simulink library "tqd"  (R2021b)
settings: Solver=VariableStepAuto  StartTime=0.0  StopTime=10.0  RelTol=1e-3
undefined symbols (not defined in the file or in its folder): ATQD_BOSEnBPSPosn_X_kph, ATQD_BOSMap_X_rpm, ATQD_BOSMap_Y_pct, ATQD_CreepBaseTqD_X_kph, ATQD_CreepBaseTqD_Y_Deg, ATQD_CreepBaseTqR_X_kph, ATQD_CreepBaseTqR_Y_Deg, ATQD_CreepBPSDisPosn_X_Deg, ATQD_CreepBPSDisPosnR_X_Deg, ATQD_CreepBPSEnPosn_X_Deg, ATQD_CreepBPSEnPosnR_X_Deg, ATQD_CreepDeltaTq_X_kph, ATQD_CreepIterm_X_kph, ATQD_CreepIterm_Y_kph, ATQD_CreepItermMaxLimit_X_pct, ATQD_CreepPreloadTime_X_kph, ATQD_CreepPreloadTq_X_kph, ATQD_CreepPreloadTq_Y_s, ATQD_CreepProtTq_X_Deg, ATQD_CreepPterm_X_kph, ATQD_ECOTqMapD_X_rpm, ATQD_ECOTqMapD_Y_pct, ATQD_NL1TqMapD_X_rpm, ATQD_NL1TqMapD_Y_pct, ATQD_NRMRrEDUSpRat_X_rpm, ATQD_NRMRrEDUSpRat_Y_Nm, ATQD_PedalMapClimbUpLim_X_rpm, ATQD_PedalMapClimbUpLim_Y_Deg, ATQD_PreLoadTq_X_s, ATQD_SL1TqMapD_X_rpm, ATQD_SL1TqMapD_Y_pct, ATQD_WhlTqCapMotGain_X_pct, ATQD_WhlTqCapMotGain_Y_mV, ENUM_ACCPEDALLOWSW_LOWIDLE, ENUM_ACCPEDALLOWSW_NOIDLE, ENUM_CHRGPLUGSTA_NONE, ENUM_CRASHSTATE_NOCRASH, ENUM_DCDCFAULTSTA_WORKING, ENUM_DRIVEMODE_ECO, ENUM_DRIVEMODE_NRM, ENUM_DRIVEMODE_SPORT, ENUM_DRIVETRAIN_AWD, ENUM_DRIVETRAIN_FWD, ENUM_DRIVETRAIN_RWD, ENUM_EBSBRKSW_PRESSED, ENUM_EBSTORQUERWQ_LIMIT, ENUM_EBSTORQUERWQ_TORQUE, ENUM_EMTRQMODE_ACCL, ENUM_EMTRQMODE_BRAKING, ENUM_EMTRQMODE_COASTING, ENUM_EPBERROR_NORMAL, ENUM_EPBSTA_APPLIED, ENUM_EPBSTA_RELEASED, ENUM_EPBSTA_UNKNOWN, ENUM_EPBSTARAW_NOTSET, ENUM_EPBSTARAW_SET, ENUM_GEARACTUALPOSN_D, ENUM_GEARACTUALPOSN_N, ENUM_GEARACTUALPOSN_P, ENUM_GEARACTUALPOSN_R ... (+201)
libraries: hcu_lib x19, simulink x12
(part 1 of 6)
settings Model: Creator=13615  LastModifiedBy=FVT22063
settings SolverCC: AlgebraicLoopSolver=TrustRegion
settings DataIOCC: SaveFormat=Array  SignalLoggingSaveFormat=ModelDataLogs  ReturnWorkspaceOutputs=off
settings OptimizationCC: BlockReduction=off  BooleanDataType=off
settings DebuggingCC: SaveWithParameterizedLinksMsg=none  UnderspecifiedInitializationDetection=Classic  MergeDetectMultiDrivingBlocksExec=none  SignalResolutionControl=TryResolveAllWithWarning
settings HardwareCC: TargetUnknown=on
settings ModelReferenceCC: PropagateSignalLabelsOutOfModel=off
settings SFSimCC: SimUseLocalCustomCode=off
settings RTWCC: RTWUseLocalCustomCode=off
settings ConfigComp: CovMetricSettings=dw  CovSaveCumulativeToWorkspaceVar=on  CovSaveSingleToWorkspaceVar=on

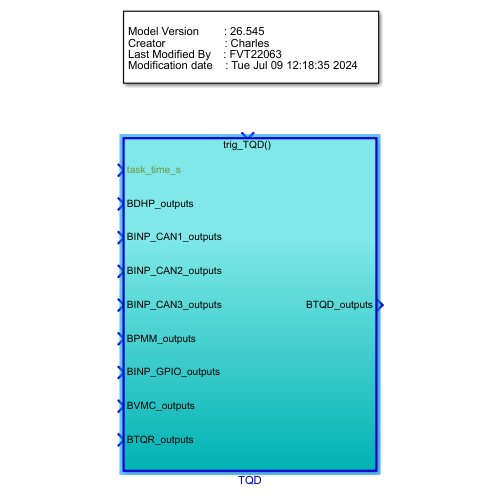
[thumbnail: Simulink's stored preview of the top-level diagram]
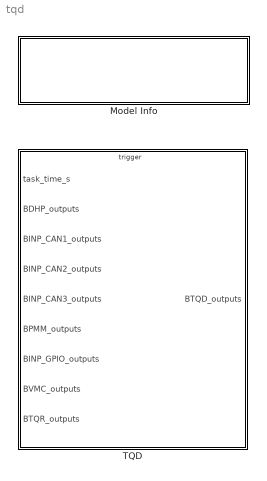
== system tqd ==
  Model Info : Subsystem  LoadFcn=slcm LoadBlock;  InitFcn=slcm('UpdateAllCMBlocksInThisModelInit')  mask(CMBlock){InitialSaveTempField=, InitialBlockCM=None, BlockCM=None, Frame=on, SaveTempField=, DisplayStringWithTags=|, MaskDisplayString=Model Version        : 26.550\nCreator                   : Charles\nLast Modified By    : FVT22063\nModification date    : Thu Aug 22 15:20:52 2024, HorizontalTextAlignment=Left, LeftAlignmentValue=0.02, SourceBlockDiagram=tqd, TagMaxNumber=20, CMTag1=, CMTag2=, CMTag3=, CMTag4=, CMTag5=, CMTag6=, CMTag7=, CMTag8=, CMTag9=, CMTag10=, CMTag11=, CMTag12=, CMTag13=, CMTag14=, CMTag15=, CMTag16=, CMTag17=, CMTag18=, CMTag19=, CMTag20=}
      mask DisplayStringWithTags=|
      | Model Version        : %<ModelVersion>
      | Creator                   : Charles
      | Last Modified By    : %<LastModifiedBy>
      | Modification date    : %<LastModificationDate>
      mask help: This block allows revision control information to be displayed within the model.
      settings: CopyFcn=slcm CopyBlock;  DeleteFcn=slcm Cancel;  PostSaveFcn=slcm('UpdateAllCMBlocksInThisModel')  NameChangeFcn=slcm Rename;  OpenFcn=slcm
      mask Display: text(str2num(LeftAlignmentValue), 0.5, MaskDisplayString, 'HorizontalAlignment', HorizontalTextAlignment)
  TQD : Subsystem
      settings: RTWSystemCode=Nonreusable function  RTWFcnNameOpts=Use subsystem name  RTWFileNameOpts=Use subsystem name

== system tqd/Model Info ==
  EmptySubsystem : Subsystem

== system tqd/TQD ==
  task_time_s : Inport
  BDHP_outputs : Inport  Port=2  OutDataTypeStr=Bus: BDHP_outputs
  BINP_CAN1_outputs : Inport  Port=3  OutDataTypeStr=Bus: BINP_CAN1_outputs
  BINP_CAN2_outputs : Inport  Port=4  OutDataTypeStr=Bus: BINP_CAN2_outputs
  BINP_CAN3_outputs : Inport  Port=5  OutDataTypeStr=Bus: BINP_CAN3_outputs
  BPMM_outputs : Inport  Port=6  OutDataTypeStr=Bus: BPMM_outputs
  BINP_GPIO_outputs : Inport  Port=7  OutDataTypeStr=Bus: BINP_GPIO_outputs
  BVMC_outputs : Inport  Port=8  OutDataTypeStr=Bus: BVMC_outputs
  BTQR_outputs : Inport  Port=9  OutDataTypeStr=Bus: BTQR_outputs  LockScale=on
  trig_TQD : TriggerPort  TriggerType=function-call  VariantControl=(inherit)
  Bus Creator : BusCreator  Inputs=97  OutDataTypeStr=Bus: BTQD_outputs  NonVirtualBus=on
  Bus Selector : BusSelector  OutputSignals=VINP_IVIPWModeReq_enum
  Bus Selector1 : BusSelector  OutputSignals=VDHP_ActAPSPosn_pct,VDHP_LowIdleAccPedal_flg
  Bus Selector2 : BusSelector  OutputSignals=VINP_FASpeed_kph,VINP_BrakePedalPos_pct,VINP_EBSBrakeSw_enum,VINP_EPBParkingBrakeSta_enum,VINP_EM1OvrCtrlMBrk_enum,VINP_EM1OvrCtrlMDriv_enum,VINP_EM1ReqTorqLimBrk_pct,VINP_EM1ReqTorqLimDriv_pct
  Bus Selector3 : BusSelector  OutputSignals=VINP_CrashSignalGPIO_flg,VINP_DrDoorSW_flg,VINP_HoodSW_flg,VINP_TailgateSW_flg,VINP_PsDoorSW_flg,VINP_RRDoorSW_flg,VINP_RLDoorSW_flg
  Bus Selector4 : BusSelector  OutputSignals=VINP_ShifterHandleCmd_enum,VINP_RrEDURotateDirction_enum,VINP_RrTMSpd_rpm,VINP_HVBPwrAvailDchrg_kW,VINP_HVBPwrAvailChrg_kW,VINP_RrRegenAvailTq_Nm,VINP_RrEDURealTMTq_Nm,VINP_HVBattErr_flg,VINP_DCDCFaultSta_enum,VINP_MCUWarnR_enum,VINP_ChrgPlugSta_enum,VINP_HVBCellVoltMax_mV,VINP_HVBCellVoltMin_mV,VINP_HVBSOH_pct,VINP_HVBattSOC_pct
  Bus Selector5 : BusSelector  OutputSignals=VVMC_EstSlope_Deg,VVMC_RWDRDCActive_enum
  Bus Selector7 : BusSelector  OutputSignals=VPMM_PowerSta_enum,VPMM_DrivetrainSelect_enum
  Bus Selector8 : BusSelector  OutputSignals=VTQR_ActualFEDUWhlTqReq_Nm,VTQR_ActualREDUWhlTqReq_Nm,VTQR_NoABSFEDUWhlTqReq_Nm,VTQR_NoABSREDUWhlTqReq_Nm,VTQR_RampREDUWhlTqReq_Nm
  Cast To Boolean{,7..8,19} (4 alike) : DataTypeConversion  OutDataTypeStr=boolean
  Cast To Boolean{11..12,31..33} (5 alike) : DataTypeConversion  OutDataTypeStr=single
  Cast To Boolean{13,16,30,35..36} (5 alike) : DataTypeConversion  OutDataTypeStr=uint8
  Data Type Conversion : DataTypeConversion  OutDataTypeStr=uint8
  Data Type Conversion{1..3,5} (4 alike) : DataTypeConversion  OutDataTypeStr=boolean
  Data Type Conversion4 : DataTypeConversion  OutDataTypeStr=uint8
  Ground{,1..2,11..13,16..18,24,32..35,37..38} (16 alike) : Ground
  TorqueDemand : Subsystem
  BTQD_outputs : Outport  OutDataTypeStr=Bus: BTQD_outputs
  wires:
  Bus Selector8/2 -> TorqueDemand/53(VTQR_ActualREDUWhlTqReq_Nm)  "<VTQR_ActualREDUWhlTqReq_Nm>"
  Bus Selector8/1 -> TorqueDemand/52(VTQR_ActualFEDUWhlTqReq_Nm)  "<VTQR_ActualFEDUWhlTqReq_Nm>"
  BTQR_outputs/1 -> Bus Selector8/1
  Bus Selector3/1 -> TorqueDemand/45(VINP_CrashSignalGPIO_flg)  "<VINP_CrashSignalGPIO_flg>"
  Bus Selector4/9 -> TorqueDemand/35(VINP_DCDCFaultSta_enum)  "<VINP_DCDCFaultSta_enum>"
  Bus Selector4/8 -> TorqueDemand/34(VINP_HVBattErr_flg)  "<VINP_HVBattErr_flg>"
  Bus Selector4/7 -> TorqueDemand/33(VINP_RrEDURealTMTq_Nm)  "<VINP_RrEDURealTMTq_Nm>"
  Bus Selector4/6 -> TorqueDemand/32(VINP_RrRegenAvailTq_Nm)  "<VINP_RrRegenAvailTq_Nm>"
  BDHP_outputs/1 -> Bus Selector1/1
  Bus Selector/1 -> TorqueDemand/26(VINP_IVIPWModeReq_enum)  "<VINP_IVIPWModeReq_enum>"
  BINP_CAN2_outputs/1 -> Bus Selector/1  "BINP_CAN2_outputs"
  Ground1/1 -> Data Type Conversion/1
  BVMC_outputs/1 -> Bus Selector5/1
  Bus Selector7/2 -> TorqueDemand/5(VPMM_DrivetrainSelect_enum)  "<VPMM_DrivetrainSelect_enum>"
  BINP_GPIO_outputs/1 -> Bus Selector3/1
  Bus Selector1/2 -> TorqueDemand/3(VDHP_LowIdleAccPedal_flg)  "<VDHP_LowIdleAccPedal_flg>"
  Bus Selector1/1 -> TorqueDemand/2(VDHP_ActAPSPosn_pct)  "<VDHP_ActAPSPosn_pct>"
  Bus Selector4/2 -> TorqueDemand/28(VINP_RrEDURotateDirction_enum)  "<VINP_RrEDURotateDirction_enum>"
  Ground/1 -> Cast To Boolean/1
  Bus Selector4/4 -> TorqueDemand/30(VINP_HVBPwrAvailDchrg_kw)  "<VINP_HVBPwrAvailDchrg_kW>"
  Bus Selector4/5 -> TorqueDemand/31(VINP_HVBPwrAvailChrg_kw)  "<VINP_HVBPwrAvailChrg_kW>"
  Bus Selector4/3 -> TorqueDemand/29(VINP_RrTMSpd_RPM)  "<VINP_RrTMSpd_rpm>"
  Bus Selector4/1 -> TorqueDemand/27(VINP_ShifterHandleCmd_enum)  "<VINP_ShifterHandleCmd_enum>"
  Bus Selector7/1 -> TorqueDemand/4(VPMM_PowerSta_enum)  "<VPMM_PowerSta_enum>"
  task_time_s/1 -> TorqueDemand/1(task_time_s)  "task_time_s"
  BINP_CAN3_outputs/1 -> Bus Selector4/1
  BINP_CAN1_outputs/1 -> Bus Selector2/1
  BPMM_outputs/1 -> Bus Selector7/1
  Bus Creator/1 -> BTQD_outputs/1  "BTQD_outputs"
  Bus Selector3/2 -> TorqueDemand/46(VINP_DrDoorSW_flg)  "<VINP_DrDoorSW_flg>"
  Bus Selector4/10 -> TorqueDemand/36(VINP_MCUWarnR_enum)  "<VINP_MCUWarnR_enum>"
  Bus Selector4/11 -> TorqueDemand/37(VINP_ChrgPlugSta_enum)  "<VINP_ChrgPlugSta_enum>"
  Bus Selector8/3 -> TorqueDemand/54(VTQR_NoABSFEDUWhlTqReq_Nm)  "<VTQR_NoABSFEDUWhlTqReq_Nm>"
  Bus Selector8/4 -> TorqueDemand/55(VTQR_NoABSREDUWhlTqReq_Nm)  "<VTQR_NoABSREDUWhlTqReq_Nm>"
  Bus Selector5/1 -> TorqueDemand/43(VVMC_EstSlope_Deg)  "<VVMC_EstSlope_Deg>"
  Bus Selector3/3 -> TorqueDemand/47(VINP_HoodSW_flg)  "<VINP_HoodSW_flg>"
  Bus Selector3/4 -> TorqueDemand/48(VINP_TailgateSW_flg)  "<VINP_TailgateSW_flg>"
  Bus Selector3/5 -> TorqueDemand/49(VINP_PsDoorSW_flg)  "<VINP_PsDoorSW_flg>"
  Bus Selector3/6 -> TorqueDemand/50(VINP_RRDoorSW_flg)  "<VINP_RRDoorSW_flg>"
  Bus Selector3/7 -> TorqueDemand/51(VINP_RLDoorSW_flg)  "<VINP_RLDoorSW_flg>"
  Bus Selector5/2 -> TorqueDemand/44(VVMC_RWDRDCActive_enum)  "<VVMC_RWDRDCActive_enum>"
  Bus Selector4/12 -> TorqueDemand/38(VINP_HVBCellVoltMax_mV)  "<VINP_HVBCellVoltMax_mV>"
  Bus Selector4/13 -> TorqueDemand/39(VINP_HVBCellVoltMin_mV)  "<VINP_HVBCellVoltMin_mV>"
  Bus Selector4/14 -> TorqueDemand/40(VINP_HVBSOH_pct)  "<VINP_HVBSOH_pct>"
  Bus Selector4/15 -> TorqueDemand/41(VINP_HVBattSOC_pct)  "<VINP_HVBattSOC_pct>"
  TorqueDemand/1(VTQD_GearActualPosn_enum) -> Bus Creator/1
  TorqueDemand/2(VTQD_ParkRequest_flg) -> Bus Creator/2
  TorqueDemand/3(VTQD_PBWLockTO_flg) -> Bus Creator/3
  TorqueDemand/4(VTQD_PBWUnlockTO_flg) -> Bus Creator/4
  TorqueDemand/5(VTQD_DriverWhlTqDem_Nm) -> Bus Creator/5
  TorqueDemand/6(VTQD_AfterAvailableTqDemFr_Nm) -> Bus Creator/6
  TorqueDemand/7(VTQD_AfterAvailableTqDemRr_Nm) -> Bus Creator/7
  TorqueDemand/8(VTQD_TqSourceFr_enum) -> Bus Creator/8
  TorqueDemand/9(VTQD_TqSourceRr_enum) -> Bus Creator/9
  TorqueDemand/10(VTQD_FrEDUAvailBrkRgnTq_Nm) -> Bus Creator/10
  TorqueDemand/11(VTQD_RrEDUAvailBrkRgnTq_Nm) -> Bus Creator/11
  TorqueDemand/12(VTQD_TqTargetShaftSpd_rpm) -> Bus Creator/12
  TorqueDemand/13(VTQD_LimpHomeAct_flg) -> Bus Creator/13
  TorqueDemand/14(VTQD_RollRegenEnable_flg) -> Bus Creator/14
  TorqueDemand/15(VTQD_EVDriveMode_enum) -> Bus Creator/15
  Bus Selector2/1 -> TorqueDemand/6(VINP_FASpeed_kph)  "<VINP_FASpeed_kph>"
  Bus Selector2/2 -> TorqueDemand/7(VINP_BrakePedalPos_pct)  "<VINP_BrakePedalPos_pct>"
  Bus Selector2/3 -> TorqueDemand/8(VINP_EBSBrakeSW_enum)  "<VINP_EBSBrakeSw_enum>"
  Bus Selector2/4 -> TorqueDemand/9(VINP_EPBParkingBrakeSta_enum)  "<VINP_EPBParkingBrakeSta_enum>"
  Ground11/1 -> Cast To Boolean7/1
  Ground12/1 -> Cast To Boolean8/1
  Ground16/1 -> Cast To Boolean11/1
  Ground17/1 -> Cast To Boolean12/1
  Ground18/1 -> Cast To Boolean13/1
  Ground13/1 -> Cast To Boolean16/1
  Ground24/1 -> Cast To Boolean19/1
  Ground32/1 -> Cast To Boolean30/1
  Ground34/1 -> Cast To Boolean32/1
  Ground35/1 -> Cast To Boolean33/1
  Ground33/1 -> Cast To Boolean31/1
  Ground37/1 -> Cast To Boolean35/1
  Ground38/1 -> Cast To Boolean36/1
  Data Type Conversion/1 -> TorqueDemand/57(VINP_PBWMotorPos_enum)  "VINP_PBWMotorPos_enum"
  Cast To Boolean/1 -> TorqueDemand/58(VDDM_LimpHomeAct_flg)  "VDDM_LimpHomeAct_flg"
  Cast To Boolean7/1 -> TorqueDemand/14(VINP_FrRBCActive_flg)  "VINP_FrRBCActive_flg"
  Cast To Boolean8/1 -> TorqueDemand/15(VINP_RrRBCActive_flg)  "VINP_RrRBCActive_flg"
  Cast To Boolean11/1 -> TorqueDemand/16(VINP_FrntAxlTrqReqBrk_Nm)  "VINP_FrntAxlTrqReqBrk_Nm"
  Cast To Boolean12/1 -> TorqueDemand/17(VINP_RearAxlTrqReqBrk_Nm)  "VINP_RearAxlTrqReqBrk_Nm"
  Cast To Boolean13/1 -> TorqueDemand/18(VINP_CrashOutputSts_enum)  "VINP_CrashOutputSts_enum"
  Cast To Boolean16/1 -> TorqueDemand/19(VINP_EPBErrSta_enum)  "VINP_EPBErrSta_enum"
  Cast To Boolean19/1 -> TorqueDemand/20(VINP_HSAActive_flg)  "VINP_HSAActive_flg"
  Cast To Boolean31/1 -> TorqueDemand/22(VINP_FrTMSpd_RPM)  "VINP_FrTMSpd_RPM"
  Cast To Boolean30/1 -> TorqueDemand/21(VINP_FrEDURotateDirction_enum)  "VINP_FrEDURotateDirction_enum"
  Cast To Boolean32/1 -> TorqueDemand/23(VINP_FrRegenAvailTq_Nm)  "VINP_FrRegenAvailTq_Nm"
  Cast To Boolean33/1 -> TorqueDemand/24(VINP_FrEDURealTMTq_Nm)  "VINP_FrEDURealTMTq_Nm"
  Cast To Boolean35/1 -> TorqueDemand/25(VINP_MCUWarnF_enum)  "VINP_MCUWarnF_enum"
  Cast To Boolean36/1 -> TorqueDemand/42(VINP_RegenMode_enum)  "VINP_RegenMode_enum"
  TorqueDemand/16(VTQD_ShiftGearPosn_enum) -> Bus Creator/16
  TorqueDemand/17(VTQD_PButtonSta_enum) -> Bus Creator/17
  TorqueDemand/18(VTQD_FrActvDmpDisabReq_flg) -> Bus Creator/18
  TorqueDemand/19(VTQD_RrActvDmpDisabReq_flg) -> Bus Creator/19
  TorqueDemand/20(VTQD_FrRgnDecrSta_flg) -> Bus Creator/20
  TorqueDemand/21(VTQD_RrRgnDecrSta_flg) -> Bus Creator/21
  TorqueDemand/22(VTQD_DriverWhlTqDemFr_Nm) -> Bus Creator/22
  TorqueDemand/23(VTQD_DriverWhlTqDemRr_Nm) -> Bus Creator/23
  TorqueDemand/24(VTQD_FrEDUActTq_Nm) -> Bus Creator/24
  TorqueDemand/25(VTQD_RrEDUActTq_Nm) -> Bus Creator/25
  TorqueDemand/26(VTQD_FrEDURolRgnTq_Nm) -> Bus Creator/26
  TorqueDemand/27(VTQD_RrEDURolRgnTq_Nm) -> Bus Creator/27
  TorqueDemand/28(VTQD_FrEDUSpd_rpm) -> Bus Creator/28
  TorqueDemand/29(VTQD_RrEDUSpd_rpm) -> Bus Creator/29
  TorqueDemand/30(VTQD_FrEDUSpdValid_flg) -> Bus Creator/30
  TorqueDemand/31(VTQD_FrEDUAvailBrkRgnTqV_flg) -> Bus Creator/31
  TorqueDemand/32(VTQD_RrEDUSpdValid_flg) -> Bus Creator/32
  TorqueDemand/33(VTQD_RrEDUAvailBrkRgnTqV_flg) -> Bus Creator/33
  TorqueDemand/34(VTQD_RgnAbnorSta_flg) -> Bus Creator/34
  TorqueDemand/35(VTQD_PTCSPermSta_flg) -> Bus Creator/35
  TorqueDemand/36(VTQD_FrRgnPermSta_flg) -> Bus Creator/36
  TorqueDemand/37(VTQD_RrRgnPermSta_flg) -> Bus Creator/37
  TorqueDemand/38(VTQD_ExternalTqAllow_flg) -> Bus Creator/38
  TorqueDemand/39(VTQD_FrIdcMin_A) -> Bus Creator/39
  TorqueDemand/40(VTQD_FrIdcMax_A) -> Bus Creator/40
  TorqueDemand/41(VTQD_FrUdcMin_V) -> Bus Creator/41
  TorqueDemand/42(VTQD_FrUdcMax_V) -> Bus Creator/42
  TorqueDemand/43(VTQD_RrIdcMin_A) -> Bus Creator/43
  TorqueDemand/44(VTQD_RrIdcMax_A) -> Bus Creator/44
  TorqueDemand/45(VTQD_RrUdcMin_V) -> Bus Creator/45
  TorqueDemand/46(VTQD_RrUdcMax_V) -> Bus Creator/46
  TorqueDemand/47(VTQD_CoordWhlTqDemFr_Nm) -> Bus Creator/47
  TorqueDemand/48(VTQD_CoordWhlTqDemRr_Nm) -> Bus Creator/48
  TorqueDemand/49(VTQD_CreepEnable_flg) -> Bus Creator/49
  TorqueDemand/50(VTQD_CrashDetd_flg) -> Bus Creator/50
  TorqueDemand/51(VTQD_DiagHCrash_flg) -> Bus Creator/51
  TorqueDemand/52(VTQD_ReBrakeLPReq_flg) -> Bus Creator/52
  TorqueDemand/53(VTQD_LowIdleAccPedal_flg) -> Bus Creator/53
  TorqueDemand/54(VTQD_ExtShftAllow_flg) -> Bus Creator/54
  TorqueDemand/55(VTQD_BOSEnable_flg) -> Bus Creator/55
  TorqueDemand/56(VTQD_CreepON_flg) -> Bus Creator/56
  TorqueDemand/57(VTQD_PreLoadHold_flg) -> Bus Creator/57
  TorqueDemand/58(VTQD_PreLoadPreEn_flg) -> Bus Creator/58
  TorqueDemand/59(VTQD_CreepPrLoadEnable_flg) -> Bus Creator/59
  TorqueDemand/60(VTQD_RDCActive_enum) -> Bus Creator/60
  TorqueDemand/61(VTQD_ExtDoorAllow_flg) -> Bus Creator/61
  TorqueDemand/62(VTQD_WhlTqCapGenFr_Nm) -> Bus Creator/62
  TorqueDemand/63(VTQD_WhlTqCapGenRr_Nm) -> Bus Creator/63
  TorqueDemand/64(VTQD_RegenMode_enum) -> Bus Creator/64
  TorqueDemand/65(VTQD_ActEMpTrq_pct) -> Bus Creator/65
  TorqueDemand/66(VTQD_ActMaxAvaEMRecpTrq_pct) -> Bus Creator/66
  TorqueDemand/67(VTQD_ActDriveDirect_enum) -> Bus Creator/67
  TorqueDemand/68(VTQD_DLEngaged_enum) -> Bus Creator/68
  TorqueDemand/69(VTQD_EMTrqModeDrvBrk_enum) -> Bus Creator/69
  TorqueDemand/70(VTQD_ActEMpTrqHrls_pct) -> Bus Creator/70
  TorqueDemand/71(VTQD_ActEMOutSftSpd_rpm) -> Bus Creator/71
  TorqueDemand/72(VTQD_DrvDemEMRtapTrq_pct) -> Bus Creator/72
  TorqueDemand/73(VTQD_SACtrlDev_enum) -> Bus Creator/73
  TorqueDemand/74(VTQD_RetSelNonEng_pct) -> Bus Creator/74
  TorqueDemand/75(VTQD_ShiftPgs_enum) -> Bus Creator/75
  TorqueDemand/76(VTQD_AccPedal1LowSW_enum) -> Bus Creator/76
  TorqueDemand/77(VTQD_AccPedalPos1_pct) -> Bus Creator/77
  TorqueDemand/78(VTQD_ParkBrakeSW_enum) -> Bus Creator/78
  TorqueDemand/79(VTQD_VCUVehSpd_kph) -> Bus Creator/79
  TorqueDemand/80(VTQD_BrakeSW_enum) -> Bus Creator/80
  TorqueDemand/81(VTQD_NFricPercTorq_pct) -> Bus Creator/81
  TorqueDemand/82(VTQD_EMParasLoss_pct) -> Bus Creator/82
  TorqueDemand/83(VTQD_EEC2MSGCnt_raw) -> Bus Creator/83
  TorqueDemand/84(VTQD_EEC2MSGCS_raw) -> Bus Creator/84
  TorqueDemand/85(VTQD_FDCCHAEBSRd4BRSta_enum) -> Bus Creator/85
  TorqueDemand/86(VTQD_FDCCHAEBSHBSwSta_enum) -> Bus Creator/86
  TorqueDemand/87(VTQD_FDCCHAEBSHHSwSta_enum) -> Bus Creator/87
  TorqueDemand/88(VTQD_FDCVCUTUpAStaSta_enum) -> Bus Creator/88
  TorqueDemand/89(VTQD_FDCVCUDACStatusSta_enum) -> Bus Creator/89
  TorqueDemand/90(VTQD_CoordTqDem_Nm) -> Bus Creator/90
  Bus Selector8/5 -> TorqueDemand/56(VTQR_RampREDUWhlTqReq_Nm)  "<VTQR_RampREDUWhlTqReq_Nm>"
  TorqueDemand/91(VTQD_FrEDUSpRat_rat) -> Bus Creator/91
  TorqueDemand/92(VTQD_RrEDUSpRat_rat) -> Bus Creator/92
  Bus Selector2/5 -> TorqueDemand/10(VINP_EM1OvrCtrlMBrk_enum)  "<VINP_EM1OvrCtrlMBrk_enum>"
  Bus Selector2/8 -> TorqueDemand/13(VINP_EM1ReqTorqLimDriv_pct)  "<VINP_EM1ReqTorqLimDriv_pct>"
  Bus Selector2/7 -> TorqueDemand/12(VINP_EM1ReqTorqLimBrk_pct)  "<VINP_EM1ReqTorqLimBrk_pct>"
  Bus Selector2/6 -> TorqueDemand/11(VINP_EM1OvrCtrlMDriv_enum)  "<VINP_EM1OvrCtrlMDriv_enum>"
  Ground2/1 -> Data Type Conversion1/1, Data Type Conversion2/1, Data Type Conversion3/1, Data Type Conversion4/1, Data Type Conversion5/1
  Data Type Conversion1/1 -> Bus Creator/93  "VTQD_EquivAccPedalSWSta_flg"
  Data Type Conversion2/1 -> Bus Creator/94  "VTQD_DriveProtEn_flg"
  Data Type Conversion3/1 -> Bus Creator/95  "VTQD_ActParkRequest_flg"
  Data Type Conversion4/1 -> Bus Creator/96  "VTQD_IVIPwrLockSta_enum"
  Data Type Conversion5/1 -> Bus Creator/97  "VTQD_OPDHoldLamp_flg"

== system tqd/Model Info/EmptySubsystem ==

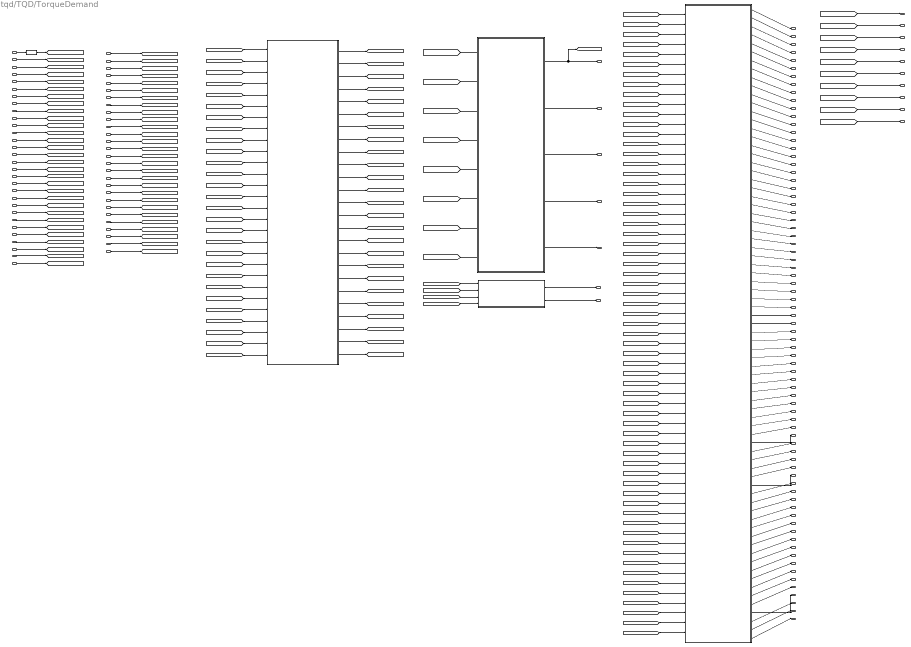
== system tqd/TQD/TorqueDemand ==
  note: Input Signals
  task_time_s : Inport
  VDHP_ActAPSPosn_pct : Inport  Port=2
  VDHP_LowIdleAccPedal_flg : Inport  Port=3
  VPMM_PowerSta_enum : Inport  Port=4
  VPMM_DrivetrainSelect_enum : Inport  Port=5
  VINP_FASpeed_kph : Inport  Port=6
  VINP_BrakePedalPos_pct : Inport  Port=7
  VINP_EBSBrakeSW_enum : Inport  Port=8
  VINP_EPBParkingBrakeSta_enum : Inport  Port=9
  VINP_EM1OvrCtrlMBrk_enum : Inport  Port=10
  VINP_EM1OvrCtrlMDriv_enum : Inport  Port=11
  VINP_EM1ReqTorqLimBrk_pct : Inport  Port=12
  VINP_EM1ReqTorqLimDriv_pct : Inport  Port=13
  VINP_FrRBCActive_flg : Inport  Port=14
  VINP_RrRBCActive_flg : Inport  Port=15
  VINP_FrntAxlTrqReqBrk_Nm : Inport  Port=16
  VINP_RearAxlTrqReqBrk_Nm : Inport  Port=17
  VINP_CrashOutputSts_enum : Inport  Port=18
  VINP_EPBErrSta_enum : Inport  Port=19
  VINP_HSAActive_flg : Inport  Port=20
  VINP_FrEDURotateDirction_enum : Inport  Port=21
  VINP_FrTMSpd_RPM : Inport  Port=22
  VINP_FrRegenAvailTq_Nm : Inport  Port=23
  VINP_FrEDURealTMTq_Nm : Inport  Port=24
  VINP_MCUWarnF_enum : Inport  Port=25
  VINP_IVIPWModeReq_enum : Inport  Port=26
  VINP_ShifterHandleCmd_enum : Inport  Port=27
  VINP_RrEDURotateDirction_enum : Inport  Port=28
  VINP_RrTMSpd_RPM : Inport  Port=29
  VINP_HVBPwrAvailDchrg_kw : Inport  Port=30
  VINP_HVBPwrAvailChrg_kw : Inport  Port=31
  VINP_RrRegenAvailTq_Nm : Inport  Port=32
  VINP_RrEDURealTMTq_Nm : Inport  Port=33
  VINP_HVBattErr_flg : Inport  Port=34
  VINP_DCDCFaultSta_enum : Inport  Port=35
  VINP_MCUWarnR_enum : Inport  Port=36
  VINP_ChrgPlugSta_enum : Inport  Port=37
  VINP_HVBCellVoltMax_mV : Inport  Port=38
  VINP_HVBCellVoltMin_mV : Inport  Port=39
  VINP_HVBSOH_pct : Inport  Port=40
  VINP_HVBattSOC_pct : Inport  Port=41
  VINP_RegenMode_enum : Inport  Port=42
  VVMC_EstSlope_Deg : Inport  Port=43
  VVMC_RWDRDCActive_enum : Inport  Port=44
  VINP_CrashSignalGPIO_flg : Inport  Port=45
  VINP_DrDoorSW_flg : Inport  Port=46
  VINP_HoodSW_flg : Inport  Port=47
  VINP_TailgateSW_flg : Inport  Port=48
  VINP_PsDoorSW_flg : Inport  Port=49
  VINP_RRDoorSW_flg : Inport  Port=50
  VINP_RLDoorSW_flg : Inport  Port=51
  VTQR_ActualFEDUWhlTqReq_Nm : Inport  Port=52
  VTQR_ActualREDUWhlTqReq_Nm : Inport  Port=53
  VTQR_NoABSFEDUWhlTqReq_Nm : Inport  Port=54
  VTQR_NoABSREDUWhlTqReq_Nm : Inport  Port=55
  VTQR_RampREDUWhlTqReq_Nm : Inport  Port=56
  VINP_PBWMotorPos_enum : Inport  Port=57
  VDDM_LimpHomeAct_flg : Inport  Port=58
  CrashDetect : Subsystem
  Data Type Conversion3 : DataTypeConversion  OutDataTypeStr=single
  ShiftModule : Subsystem
      settings: AttributesFormatString=Priority%<Priority>
  Signal_convert : Subsystem
  TorqueModule : Subsystem
      settings: AttributesFormatString=Priority%<Priority>
  VTQD_GearActualPosn_enum : Outport
  VTQD_ParkRequest_flg : Outport  Port=2
  VTQD_PBWLockTO_flg : Outport  Port=3
  VTQD_PBWUnlockTO_flg : Outport  Port=4
  VTQD_DriverWhlTqDem_Nm : Outport  Port=5
  VTQD_AfterAvailableTqDemFr_Nm : Outport  Port=6
  VTQD_AfterAvailableTqDemRr_Nm : Outport  Port=7
  VTQD_TqSourceFr_enum : Outport  Port=8
  VTQD_TqSourceRr_enum : Outport  Port=9
  VTQD_FrEDUAvailBrkRgnTq_Nm : Outport  Port=10
  VTQD_RrEDUAvailBrkRgnTq_Nm : Outport  Port=11
  VTQD_TqTargetShaftSpd_rpm : Outport  Port=12
  VTQD_LimpHomeAct_flg : Outport  Port=13
  VTQD_RollRegenEnable_flg : Outport  Port=14
  VTQD_EVDriveMode_enum : Outport  Port=15
  VTQD_ShiftGearPosn_enum : Outport  Port=16
  VTQD_PButtonSta_enum : Outport  Port=17
  VTQD_FrActvDmpDisabReq_flg : Outport  Port=18
  VTQD_RrActvDmpDisabReq_flg : Outport  Port=19
  VTQD_FrRgnDecrSta_flg : Outport  Port=20
  VTQD_RrRgnDecrSta_flg : Outport  Port=21
  VTQD_DriverWhlTqDemFr_Nm : Outport  Port=22
  VTQD_DriverWhlTqDemRr_Nm : Outport  Port=23
  VTQD_FrEDUActTq_Nm : Outport  Port=24
  VTQD_RrEDUActTq_Nm : Outport  Port=25
  VTQD_FrEDURolRgnTq_Nm : Outport  Port=26
  VTQD_RrEDURolRgnTq_Nm : Outport  Port=27
  VTQD_FrEDUSpd_rpm : Outport  Port=28
  VTQD_RrEDUSpd_rpm : Outport  Port=29
  VTQD_FrEDUSpdValid_flg : Outport  Port=30
  VTQD_FrEDUAvailBrkRgnTqV_flg : Outport  Port=31
  VTQD_RrEDUSpdValid_flg : Outport  Port=32
  VTQD_RrEDUAvailBrkRgnTqV_flg : Outport  Port=33
  VTQD_RgnAbnorSta_flg : Outport  Port=34
  VTQD_PTCSPermSta_flg : Outport  Port=35
  VTQD_FrRgnPermSta_flg : Outport  Port=36
  VTQD_RrRgnPermSta_flg : Outport  Port=37
  VTQD_ExternalTqAllow_flg : Outport  Port=38
  VTQD_FrIdcMin_A : Outport  Port=39
  VTQD_FrIdcMax_A : Outport  Port=40
  VTQD_FrUdcMin_V : Outport  Port=41
  VTQD_FrUdcMax_V : Outport  Port=42
  VTQD_RrIdcMin_A : Outport  Port=43
  VTQD_RrIdcMax_A : Outport  Port=44
  VTQD_RrUdcMin_V : Outport  Port=45
  VTQD_RrUdcMax_V : Outport  Port=46
  VTQD_CoordWhlTqDemFr_Nm : Outport  Port=47
  VTQD_CoordWhlTqDemRr_Nm : Outport  Port=48
  VTQD_CreepEnable_flg : Outport  Port=49
  VTQD_CrashDetd_flg : Outport  Port=50
  VTQD_DiagHCrash_flg : Outport  Port=51
  VTQD_ReBrakeLPReq_flg : Outport  Port=52
  VTQD_LowIdleAccPedal_flg : Outport  Port=53
  VTQD_ExtShftAllow_flg : Outport  Port=54
  VTQD_BOSEnable_flg : Outport  Port=55
  VTQD_CreepON_flg : Outport  Port=56
  VTQD_PreLoadHold_flg : Outport  Port=57
  VTQD_PreLoadPreEn_flg : Outport  Port=58
  VTQD_CreepPrLoadEnable_flg : Outport  Port=59
  VTQD_RDCActive_enum : Outport  Port=60
  VTQD_ExtDoorAllow_flg : Outport  Port=61
  VTQD_WhlTqCapGenFr_Nm : Outport  Port=62
  VTQD_WhlTqCapGenRr_Nm : Outport  Port=63
  VTQD_RegenMode_enum : Outport  Port=64
  VTQD_ActEMpTrq_pct : Outport  Port=65
  VTQD_ActMaxAvaEMRecpTrq_pct : Outport  Port=66
  VTQD_ActDriveDirect_enum : Outport  Port=67
  VTQD_DLEngaged_enum : Outport  Port=68
  VTQD_EMTrqModeDrvBrk_enum : Outport  Port=69
  VTQD_ActEMpTrqHrls_pct : Outport  Port=70
  VTQD_ActEMOutSftSpd_rpm : Outport  Port=71
  VTQD_DrvDemEMRtapTrq_pct : Outport  Port=72
  VTQD_SACtrlDev_enum : Outport  Port=73
  VTQD_RetSelNonEng_pct : Outport  Port=74
  VTQD_ShiftPgs_enum : Outport  Port=75
  VTQD_AccPedal1LowSW_enum : Outport  Port=76
  VTQD_AccPedalPos1_pct : Outport  Port=77
  VTQD_ParkBrakeSW_enum : Outport  Port=78
  VTQD_VCUVehSpd_kph : Outport  Port=79
  VTQD_BrakeSW_enum : Outport  Port=80
  VTQD_NFricPercTorq_pct : Outport  Port=81
  VTQD_EMParasLoss_pct : Outport  Port=82
  VTQD_EEC2MSGCnt_raw : Outport  Port=83
  VTQD_EEC2MSGCS_raw : Outport  Port=84
  VTQD_FDCCHAEBSRd4BRSta_enum : Outport  Port=85
  VTQD_FDCCHAEBSHBSwSta_enum : Outport  Port=86
  VTQD_FDCCHAEBSHHSwSta_enum : Outport  Port=87
  VTQD_FDCVCUTUpAStaSta_enum : Outport  Port=88
  VTQD_FDCVCUDACStatusSta_enum : Outport  Port=89
  VTQD_CoordTqDem_Nm : Outport  Port=90
  VTQD_FrEDUSpRat_rat : Outport  Port=91
  VTQD_RrEDUSpRat_rat : Outport  Port=92
  wires:
  VINP_FrTMSpd_RPM/1 -> [VINP_FrTMSpd_rpm]
  VDHP_ActAPSPosn_pct/1 -> [VDHP_ActAPSPosn_pct]
  VPMM_PowerSta_enum/1 -> [VPMM_PowerSta_enum]
  task_time_s/1 -> Data Type Conversion3/1
  VINP_FASpeed_kph/1 -> [VINP_VehSpeed_kph]
  VINP_EBSBrakeSW_enum/1 -> [VINP_EBSBrakeSW_enum]
  VINP_ShifterHandleCmd_enum/1 -> [VINP_ShifterHandleCmd_enum]
  VDHP_LowIdleAccPedal_flg/1 -> [VDHP_LowIdleAccPedal_flg]
  VINP_PBWMotorPos_enum/1 -> [VINP_PBWMotorPos_enum]
  Signal_convert/8(VTQD_TqTargetShaftSpd_rpm) -> [VTQD_TqTargetShaftSpd_rpm]
  Signal_convert/2(VTQD_RollRegenDisable_flg) -> [VTQD_RollRegenDisableReq_flg]
  Signal_convert/5(VTQD_ActBPSPosn_pct) -> [VTQD_ActBPSPosn_pct]
  Signal_convert/11(VTQD_EVDriveMode_enum) -> [VTQD_EVDriveMode_enum]
  Signal_convert/10(VTQD_LimpHomeAct_flg) -> [VTQD_LimpHomeAct_flg]
  Signal_convert/12(VTQD_CreepON_flg) -> [VTQD_CreepON_flg]
  [VTQD_TMRotateDirction_enum] -> ShiftModule/7(VTQD_TMRotateDirction_enum)
  ShiftModule/4(VTQD_PBWUnlockTO_flg) -> VTQD_PBWUnlockTO_flg/1
  [VINP_VehSpeed_kph] -> ShiftModule/3(VINP_VehSpeed_kph)
  [VPMM_PowerSta_enum] -> ShiftModule/5(VPMM_PowerSta_enum)
  [task_time_s] -> ShiftModule/1(task_time_s)
  [VTQD_BrkSwSta_flg] -> ShiftModule/4(VTQD_BrkSwSta_flg)
  ShiftModule/2(VTQD_ParkRequest_flg) -> VTQD_ParkRequest_flg/1
  [VINP_ShifterHandleCmd_enum] -> ShiftModule/2(VINP_ShifterHandleCmd_enum)
  ShiftModule/3(VTQD_PBWLockTO_flg) -> VTQD_PBWLockTO_flg/1
  [VINP_PBWMotorPos_enum] -> ShiftModule/6(VINP_PBWMotorPos_enum)
  ShiftModule/1(VTQD_GearActualPosn_enum) -> [VTQD_GearActualPosn_enum], VTQD_GearActualPosn_enum/1
  [VTQD_RollRegenDisableReq_flg] -> TorqueModule/3(VTQD_RollRegenDisableReq_flg)
  [VTQD_GearActualPosn_enum] -> TorqueModule/4(VTQD_GearActualPosn_enum)
  [VTQD_CreepON_flg] -> TorqueModule/5(VTQD_CreepON_flg)
  [VTQD_BrkSwSta_flg] -> TorqueModule/6(VTQD_BrkSwSta_flg)
  [VINP_FrntAxlTrqReqBrk_Nm] -> TorqueModule/18(VINP_FrntAxlTrqReqBrk_Nm)
  [VINP_RearAxlTrqReqBrk_Nm] -> TorqueModule/19(VINP_RearAxlTrqReqBrk_Nm)
  [VTQD_LimpHomeAct_flg] -> TorqueModule/7(VTQD_LimpHomeAct_flg)
  [VINP_VehSpeed_kph] -> TorqueModule/10(VINP_VehSpeed_kph)
  [VTQD_TqTargetShaftSpd_rpm] -> TorqueModule/11(VTQD_TqTargetShaftSpd_rpm)
  [VTQD_ActBPSPosn_pct] -> TorqueModule/15(VTQD_ActBPSPosn_pct)
  VINP_HVBPwrAvailDchrg_kw/1 -> [VINP_HVBPwrAvailDchrg_kw]
  VINP_HVBPwrAvailChrg_kw/1 -> [VINP_HVBPwrAvailChrg_kw]
  [VINP_HVBPwrAvailDchrg_kw] -> TorqueModule/20(VINP_HVBPwrAvailDchrg_kw)
  [VINP_HVBPwrAvailChrg_kw] -> TorqueModule/21(VINP_HVBPwrAvailChrg_kw)
  VDDM_LimpHomeAct_flg/1 -> [VDDM_LimpHomeAct_flg]
  [VDDM_LimpHomeAct_flg] -> Signal_convert/11(VDDM_LimpHomeAct_flg)
  VINP_FrRBCActive_flg/1 -> [VINP_FrRBCActive_flg]
  VINP_FrntAxlTrqReqBrk_Nm/1 -> [VINP_FrntAxlTrqReqBrk_Nm]
  VINP_RearAxlTrqReqBrk_Nm/1 -> [VINP_RearAxlTrqReqBrk_Nm]
  VINP_BrakePedalPos_pct/1 -> [VINP_BrkPedalPos_pct]
  [VINP_EBSBrakeSW_enum] -> Signal_convert/4(VINP_EBSBrakeSW_enum)
  [VINP_BrkPedalPos_pct] -> Signal_convert/5(VINP_BrkPedalPos_pct)
  [VTQD_TqTargetShaftSpd_rpm] -> VTQD_TqTargetShaftSpd_rpm/1
  [VTQD_LowIdleAccPedal_flg] -> TorqueModule/1(VTQD_LowIdleAccPedal_flg)
  [VPMM_DrivetrainSelect_enum] -> TorqueModule/2(VPMM_DrivetrainSelect_enum)
  VINP_RrTMSpd_RPM/1 -> [VINP_RrTMSpd_rpm]
  [VPMM_DrivetrainSelect_enum] -> Signal_convert/8(VPMM_DrivetrainSelect_enum)
  VPMM_DrivetrainSelect_enum/1 -> [VPMM_DrivetrainSelect_enum]
  [VDHP_ActAPSPosn_pct] -> Signal_convert/3(VDHP_ActAPSPosn_pct)
  Signal_convert/3(VTQD_ActAPSPosn_pct) -> [VTQD_ActAPSPosn_pct]
  [VTQD_ActAPSPosn_pct] -> TorqueModule/14(VTQD_ActAPSPosn_pct)
  [VTQD_GearActualPosn_enum] -> Signal_convert/1(VTQD_GearActualPosn_enum)
  [VINP_FrTMSpd_rpm] -> Signal_convert/6(VINP_FrTMSpd_rpm)
  [VINP_RrTMSpd_rpm] -> Signal_convert/7(VINP_RrTMSpd_rpm)
  VINP_FrEDURotateDirction_enum/1 -> [VINP_FrEDURotateDirction_enum]
  VINP_RrEDURotateDirction_enum/1 -> [VINP_RrEDURotateDirction_enum]
  [VINP_RrEDURotateDirction_enum] -> Signal_convert/10(VINP_RrEDURotateDirction_enum)
  [VINP_FrEDURotateDirction_enum] -> Signal_convert/9(VINP_FrEDURotateDirction_enum)
  Signal_convert/6(VTQD_FrShaftSpd_rpm) -> [VTQD_FrShaftSpd_rpm]
  Signal_convert/7(VTQD_RrShaftSpd_rpm) -> [VTQD_RrShaftSpd_rpm]
  Signal_convert/9(VTQD_TMRotateDirction_enum) -> [VTQD_TMRotateDirction_enum]
  Signal_convert/4(VTQD_BrkSwSta_flg) -> [VTQD_BrkSwSta_flg]
  [VTQD_FrShaftSpd_rpm] -> TorqueModule/12(VTQD_FrShaftSpd_rpm)
  [VTQD_RrShaftSpd_rpm] -> TorqueModule/13(VTQD_RrShaftSpd_rpm)
  Signal_convert/1(VTQD_LowIdleAccPedal_flg) -> [VTQD_LowIdleAccPedal_flg]
  [VDHP_LowIdleAccPedal_flg] -> Signal_convert/2(VDHP_LowIdleAccPedal_flg)
  [VTQD_LimpHomeAct_flg] -> VTQD_LimpHomeAct_flg/1
  [VTQD_EVDriveMode_enum] -> VTQD_EVDriveMode_enum/1
  Signal_convert/13(VTQD_ShiftGearPosn_enum) -> [VTQD_ShiftGearPosn_enum]
  [VTQD_ShiftGearPosn_enum] -> VTQD_ShiftGearPosn_enum/1
  ShiftModule/5(VTQD_PButtonSta_enum) -> VTQD_PButtonSta_enum/1
  [VINP_VehSpeed_kph] -> Signal_convert/12(VINP_VehSpeed_kph)
  Signal_convert/14(VTQD_FrActvDmpDisabReq_flg) -> [VTQD_FrActvDmpDisabReq_flg]
  Signal_convert/15(VTQD_RrActvDmpDisabReq_flg) -> [VTQD_RrActvDmpDisabReq_flg]
  [VTQD_FrActvDmpDisabReq_flg] -> VTQD_FrActvDmpDisabReq_flg/1
  [VTQD_RrActvDmpDisabReq_flg] -> VTQD_RrActvDmpDisabReq_flg/1
  VINP_RrRBCActive_flg/1 -> [VINP_RrRBCActive_flg]
  [VINP_FrRBCActive_flg] -> TorqueModule/16(VINP_FrRBCActive_flg)
  [VINP_RrRBCActive_flg] -> TorqueModule/17(VINP_RrRBCActive_flg)
  VINP_RrRegenAvailTq_Nm/1 -> [VINP_RrRegenAvailTq_Nm]
  VINP_FrEDURealTMTq_Nm/1 -> [VINP_FrEDURealTMTq_Nm]
  VINP_FrRegenAvailTq_Nm/1 -> [VINP_FrRegenAvailTq_Nm]
  VINP_RrEDURealTMTq_Nm/1 -> [VINP_RrEDURealTMTq_Nm]
  [VINP_FrRegenAvailTq_Nm] -> TorqueModule/22(VINP_FrRegenAvailTq_Nm)
  [VINP_RrRegenAvailTq_Nm] -> TorqueModule/23(VINP_RrRegenAvailTq_Nm)
  [VINP_FrTMSpd_rpm] -> TorqueModule/24(VINP_FrTMSpd_RPM)
  [VINP_RrTMSpd_rpm] -> TorqueModule/25(VINP_RrTMSpd_RPM)
  [VINP_FrEDURealTMTq_Nm] -> TorqueModule/26(VINP_FrEDURealTMTq_Nm)
  [VINP_RrEDURealTMTq_Nm] -> TorqueModule/27(VINP_RrEDURealTMTq_Nm)
  Signal_convert/16(VTQD_MCUReady4Ext_flg) -> [VTQD_MCUReady4Ext_flg]
  [VPMM_PowerSta_enum] -> TorqueModule/28(VPMM_PwrSta_enum)
  [VTQD_MCUReady4Ext_flg] -> TorqueModule/29(VTQD_MCUReady4Ext_flg)
  VINP_DCDCFaultSta_enum/1 -> [VINP_DCDCFaultSta_enum]
  VINP_HVBattErr_flg/1 -> [VINP_HVBattErr_flg]
  [VINP_HVBattErr_flg] -> TorqueModule/30(VINP_HVBattErr_flg)
  [VINP_DCDCFaultSta_enum] -> TorqueModule/31(VINP_DCDCFaultSta_enum)
  [VTQD_TMRotateDirction_enum] -> TorqueModule/32(VTQD_TMRotateDirction_enum)
  VINP_IVIPWModeReq_enum/1 -> [VINP_IVIPWModeReq_enum]
  VINP_RegenMode_enum/1 -> [VINP_RegenMode_enum]
  [VTQD_EVDriveMode_enum] -> TorqueModule/8(VTQD_EVDriveMode_enum)
  [VTQD_RegenMode_enum] -> TorqueModule/9(VTQD_RegenMode_enum)
  TorqueModule/1(VTQD_DriverWhlTqDem_Nm) -> VTQD_DriverWhlTqDem_Nm/1
  TorqueModule/2(VTQD_TqSourceFr_enum) -> VTQD_TqSourceFr_enum/1
  TorqueModule/3(VTQD_TqSourceRr_enum) -> VTQD_TqSourceRr_enum/1  "VTQD_TqSourceRr_enum"
  TorqueModule/4(VTQD_RollRegenEnable_flg) -> VTQD_RollRegenEnable_flg/1
  TorqueModule/6(VTQD_AfterAvailableTqDemRr_Nm) -> VTQD_AfterAvailableTqDemRr_Nm/1
  TorqueModule/7(VTQD_FrEDUAvailBrkRgnTq_Nm) -> VTQD_FrEDUAvailBrkRgnTq_Nm/1
  TorqueModule/8(VTQD_RrEDUAvailBrkRgnTq_Nm) -> VTQD_RrEDUAvailBrkRgnTq_Nm/1
  TorqueModule/9(VTQD_FrRgnDecrSta_flg) -> VTQD_FrRgnDecrSta_flg/1
  TorqueModule/10(VTQD_RrRgnDecrSta_flg) -> VTQD_RrRgnDecrSta_flg/1
  TorqueModule/11(VTQD_FrEDUActTq_Nm) -> VTQD_FrEDUActTq_Nm/1
  TorqueModule/12(VTQD_RrEDUActTq_Nm) -> VTQD_RrEDUActTq_Nm/1
  TorqueModule/13(VTQD_FrEDURolRgnTq_Nm) -> VTQD_FrEDURolRgnTq_Nm/1
  TorqueModule/14(VTQD_RrEDURolRgnTq_Nm) -> VTQD_RrEDURolRgnTq_Nm/1
  TorqueModule/15(VTQD_FrEDUSpd_rpm) -> VTQD_FrEDUSpd_rpm/1
  TorqueModule/16(VTQD_RrEDUSpd_rpm) -> VTQD_RrEDUSpd_rpm/1
  TorqueModule/17(VTQD_FrEDUSpdValid_flg) -> VTQD_FrEDUSpdValid_flg/1
  TorqueModule/18(VTQD_FrEDUAvailBrkRgnTqV_flg) -> VTQD_FrEDUAvailBrkRgnTqV_flg/1
  TorqueModule/19(VTQD_RrEDUSpdValid_flg) -> VTQD_RrEDUSpdValid_flg/1
  TorqueModule/20(VTQD_RrEDUAvailBrkRgnTqV_flg) -> VTQD_RrEDUAvailBrkRgnTqV_flg/1
  TorqueModule/21(VTQD_RgnAbnorSta_flg) -> VTQD_RgnAbnorSta_flg/1
  TorqueModule/22(VTQD_PTCSPermSta_flg) -> VTQD_PTCSPermSta_flg/1
  TorqueModule/23(VTQD_FrRgnPermSta_flg) -> VTQD_FrRgnPermSta_flg/1
  TorqueModule/24(VTQD_RrRgnPermSta_flg) -> VTQD_RrRgnPermSta_flg/1
  TorqueModule/25(VTQD_DriverWhlTqDemFr_Nm) -> VTQD_DriverWhlTqDemFr_Nm/1
  TorqueModule/26(VTQD_DriverWhlTqDemRr_Nm) -> VTQD_DriverWhlTqDemRr_Nm/1
  TorqueModule/27(VTQD_ExternalTqAllow_flg) -> VTQD_ExternalTqAllow_flg/1
  TorqueModule/28(VTQD_FrIdcMin_A) -> VTQD_FrIdcMin_A/1
  TorqueModule/29(VTQD_FrIdcMax_A) -> VTQD_FrIdcMax_A/1
  TorqueModule/30(VTQD_FrUdcMin_V) -> VTQD_FrUdcMin_V/1
  TorqueModule/31(VTQD_FrUdcMax_V) -> VTQD_FrUdcMax_V/1
  TorqueModule/32(VTQD_RrIdcMin_A) -> VTQD_RrIdcMin_A/1
  TorqueModule/33(VTQD_RrIdcMax_A) -> VTQD_RrIdcMax_A/1
  TorqueModule/34(VTQD_RrUdcMin_V) -> VTQD_RrUdcMin_V/1
  TorqueModule/35(VTQD_RrUdcMax_V) -> VTQD_RrUdcMax_V/1
  TorqueModule/36(VTQD_CoordWhlTqDemFr_Nm) -> VTQD_CoordWhlTqDemFr_Nm/1
  TorqueModule/37(VTQD_CoordWhlTqDemRr_Nm) -> VTQD_CoordWhlTqDemRr_Nm/1
  TorqueModule/38(VTQD_CreepEnable_flg) -> VTQD_CreepEnable_flg/1
  [VINP_IVIPWModeReq_enum] -> Signal_convert/13(VINP_IVIPWModeReq_enum)
  VINP_CrashSignalGPIO_flg/1 -> [VINP_CrashSignalGPIO_flg]
  VINP_CrashOutputSts_enum/1 -> [VINP_CrashOutputSts_enum]
  [VPMM_PowerSta_enum] -> CrashDetect/1(VPMM_PowerSta_enum)
  [VINP_CrashSignalGPIO_flg] -> CrashDetect/2(VINP_CrashSignalGPIO_flg)
  [VINP_CrashOutputSts_enum] -> CrashDetect/3(VINP_CrashOutputSts_enum)
  [task_time_s] -> CrashDetect/4(task_time_s)
  CrashDetect/1(VTQD_CrashDetd_flg) -> VTQD_CrashDetd_flg/1  "VTQD_CrashDetd_flg"
  CrashDetect/2(VTQD_DiagHCrash_flg) -> VTQD_DiagHCrash_flg/1  "VTQD_DiagHCrash_flg"
  TorqueModule/39(VTQD_ReBrakeLPReq_flg) -> VTQD_ReBrakeLPReq_flg/1
  VTQR_ActualFEDUWhlTqReq_Nm/1 -> [VTQR_ActualFEDUWhlTqReq_Nm]
  VTQR_ActualREDUWhlTqReq_Nm/1 -> [VTQR_ActualREDUWhlTqReq_Nm]
  [VTQR_ActualFEDUWhlTqReq_Nm] -> TorqueModule/33(VTQR_ActualFEDUWhlTqReq_Nm)
  [VTQR_ActualREDUWhlTqReq_Nm] -> TorqueModule/34(VTQR_ActualREDUWhlTqReq_Nm)
  [VTQD_RDCActive_enum] -> TorqueModule/35(VTQD_RDCActive_enum)
  VINP_EPBErrSta_enum/1 -> [VINP_EPBErrSta_enum]
  VINP_EPBParkingBrakeSta_enum/1 -> [VINP_EPBParkingBrakeSta_enum]
  [task_time_s] -> TorqueModule/36(task_time_s)
  TorqueModule/40(VTQD_BOSEnable_flg) -> VTQD_BOSEnable_flg/1
  VINP_HSAActive_flg/1 -> [VINP_HSAActive_flg]
  VTQR_NoABSREDUWhlTqReq_Nm/1 -> [VTQR_NoABSREDUWhlTqReq_Nm]
  VTQR_NoABSFEDUWhlTqReq_Nm/1 -> [VTQR_NoABSFEDUWhlTqReq_Nm]
  VINP_DrDoorSW_flg/1 -> [VINP_DrDoorSW_flg]
  VINP_MCUWarnF_enum/1 -> [VINP_MCUWarnF_enum]
  VINP_MCUWarnR_enum/1 -> [VINP_MCUWarnR_enum]
  VINP_ChrgPlugSta_enum/1 -> [VINP_ChrgPlugSta_enum]
  [VINP_MCUWarnF_enum] -> Signal_convert/14(VINP_MCUWarnF_enum)
  [VINP_FrEDURealTMTq_Nm] -> Signal_convert/16(VINP_FrEDURealTMTq_Nm)
  [VINP_RrEDURealTMTq_Nm] -> Signal_convert/17(VINP_RrEDURealTMTq_Nm)
  [VINP_MCUWarnR_enum] -> Signal_convert/15(VINP_MCUWarnR_enum)
  [VINP_HSAActive_flg] -> TorqueModule/37(VINP_HSAActive_flg)
  [VTQR_NoABSFEDUWhlTqReq_Nm] -> TorqueModule/38(VTQR_NoABSFEDUWhlTqReq_Nm)
  [VTQR_NoABSREDUWhlTqReq_Nm] -> TorqueModule/39(VTQR_NoABSREDUWhlTqReq_Nm)
  [VINP_EPBErrSta_enum] -> TorqueModule/40(VINP_EPBErrSta_enum)
  [VINP_MCUWarnF_enum] -> TorqueModule/41(VINP_MCUWarnF_enum)
  [VINP_MCUWarnR_enum] -> TorqueModule/42(VINP_MCUWarnR_enum)
  [VINP_ChrgPlugSta_enum] -> ShiftModule/8(VINP_ChrgPlugSta_enum)
  TorqueModule/41(VTQD_ExtShftAllow_flg) -> VTQD_ExtShftAllow_flg/1
  [VINP_RegenMode_enum] -> Signal_convert/18(VINP_RegenMode_enum)
  TorqueModule/42(VTQD_PreLoadHold_flg) -> VTQD_PreLoadHold_flg/1
  TorqueModule/43(VTQD_PreLoadPreEn_flg) -> VTQD_PreLoadPreEn_flg/1
  [VINP_FrntAxlTrqReqBrk_Nm] -> Signal_convert/19(VINP_FrntAxlTrqReqBrk_Nm)
  [VINP_RearAxlTrqReqBrk_Nm] -> Signal_convert/20(VINP_RearAxlTrqReqBrk_Nm)
  [VINP_FrRBCActive_flg] -> Signal_convert/21(VINP_FrRBCActive_flg)
  [VINP_RrRBCActive_flg] -> Signal_convert/22(VINP_RrRBCActive_flg)
  TorqueModule/44(VTQD_CreepPrLoadEnable_flg) -> VTQD_CreepPrLoadEnable_flg/1
  Signal_convert/17(VTQD_RDCActive_enum) -> [VTQD_RDCActive_enum]
  VVMC_EstSlope_Deg/1 -> [VVMC_EstSlope_Deg]
  [VVMC_EstSlope_Deg] -> TorqueModule/43(VVMC_EstSlope_Deg)
  [VVMC_RWDRDCActive_enum] -> Signal_convert/23(VVMC_RWDRDCActive_enum)
  [VINP_DrDoorSW_flg] -> TorqueModule/44(VINP_DrDoorSW_flg)
  [VINP_PsDoorSW_flg] -> TorqueModule/45(VINP_PsDoorSW_flg)
  [VINP_RRDoorSW_flg] -> TorqueModule/46(VINP_RRDoorSW_flg)
  [VINP_RLDoorSW_flg] -> TorqueModule/47(VINP_RLDoorSW_flg)
  [VINP_HoodSW_flg] -> TorqueModule/48(VINP_HoodSW_flg)
  [VINP_TailgateSW_flg] -> TorqueModule/49(VINP_TailgateSW_flg)
  [VTQD_EPBSta_enum] -> TorqueModule/50(VTQD_EPBSta_enum)
  TorqueModule/45(VTQD_ExtDoorAllow_flg) -> VTQD_ExtDoorAllow_flg/1
  VINP_RLDoorSW_flg/1 -> [VINP_RLDoorSW_flg]
  VINP_HoodSW_flg/1 -> [VINP_HoodSW_flg]
  VINP_PsDoorSW_flg/1 -> [VINP_PsDoorSW_flg]
  VINP_TailgateSW_flg/1 -> [VINP_TailgateSW_flg]
  VINP_RRDoorSW_flg/1 -> [VINP_RRDoorSW_flg]
  VVMC_RWDRDCActive_enum/1 -> [VVMC_RWDRDCActive_enum]
  TorqueModule/5(VTQD_AfterAvailableTqDemFr_Nm) -> VTQD_AfterAvailableTqDemFr_Nm/1
  VINP_HVBCellVoltMax_mV/1 -> [VINP_HVBCellVoltMax_mV]
  VINP_HVBCellVoltMin_mV/1 -> [VINP_HVBCellVoltMin_mV]
  VINP_HVBSOH_pct/1 -> [VINP_HVBSOH_pct]
  [VINP_HVBCellVoltMax_mV] -> TorqueModule/51(VINP_HVBCellVoltMax_mV)
  [VINP_HVBCellVoltMin_mV] -> TorqueModule/52(VINP_HVBCellVoltMin_mV)
  [VINP_HVBSOH_pct] -> TorqueModule/53(VINP_HVBSOH_pct)
  TorqueModule/46(VTQD_WhlTqCapGenFr_Nm) -> VTQD_WhlTqCapGenFr_Nm/1
  TorqueModule/47(VTQD_WhlTqCapGenRr_Nm) -> VTQD_WhlTqCapGenRr_Nm/1
  [VINP_HVBattSOC_pct] -> TorqueModule/54(VINP_HVBattSOC_pct)
  VINP_HVBattSOC_pct/1 -> [VINP_HVBattSOC_pct]
  Signal_convert/18(VTQD_RegenMode_enum) -> [VTQD_RegenMode_enum]
  TorqueModule/50(VTQD_ActDriveDirect_enum) -> VTQD_ActDriveDirect_enum/1
  TorqueModule/51(VTQD_DLEngaged_enum) -> VTQD_DLEngaged_enum/1
  TorqueModule/48(VTQD_ActEMpTrq_pct) -> VTQD_ActEMpTrq_pct/1
  TorqueModule/49(VTQD_ActMaxAvaEMRecpTrq_pct) -> VTQD_ActMaxAvaEMRecpTrq_pct/1
  Signal_convert/19(VTQD_EPBSta_enum) -> [VTQD_EPBSta_enum]
  Data Type Conversion3/1 -> [task_time_s]  "task_time_s"
  [VINP_EPBParkingBrakeSta_enum] -> Signal_convert/24(VINP_EPBParkingBrakeSta_enum)
  TorqueModule/52(VTQD_EMTrqModeDrvBrk_enum) -> VTQD_EMTrqModeDrvBrk_enum/1
  TorqueModule/53(VTQD_ActEMpTrqHrls_pct) -> VTQD_ActEMpTrqHrls_pct/1
  TorqueModule/54(VTQD_ActEMOutSftSpd_rpm) -> VTQD_ActEMOutSftSpd_rpm/1
  TorqueModule/55(VTQD_DrvDemEMRtapTrq_pct) -> VTQD_DrvDemEMRtapTrq_pct/1
  TorqueModule/56(VTQD_SACtrlDev_enum) -> VTQD_SACtrlDev_enum/1
  TorqueModule/57(VTQD_RetSelNonEng_pct) -> VTQD_RetSelNonEng_pct/1
  TorqueModule/58(VTQD_ShiftPgs_enum) -> VTQD_ShiftPgs_enum/1
  TorqueModule/59(VTQD_AccPedal1LowSW_enum) -> VTQD_AccPedal1LowSW_enum/1
  TorqueModule/60(VTQD_AccPedalPos1_pct) -> VTQD_AccPedalPos1_pct/1
  TorqueModule/61(VTQD_ParkBrakeSW_enum) -> VTQD_ParkBrakeSW_enum/1
  TorqueModule/62(VTQD_VCUVehSpd_kph) -> VTQD_VCUVehSpd_kph/1
  TorqueModule/63(VTQD_BrakeSW_enum) -> VTQD_BrakeSW_enum/1
  TorqueModule/64(VTQD_NFricPercTorq_pct) -> VTQD_NFricPercTorq_pct/1
  TorqueModule/65(VTQD_EMParasLoss_pct) -> VTQD_EMParasLoss_pct/1
  [VINP_EBSBrakeSW_enum] -> TorqueModule/55(VINP_EBSBrakeSW_enum)
  [VINP_EPBParkingBrakeSta_enum] -> TorqueModule/56(VINP_EPBParkingBrakeSta_enum)
  [VTQD_LowIdleAccPedal_flg] -> VTQD_LowIdleAccPedal_flg/1
  [VTQD_CreepON_flg] -> VTQD_CreepON_flg/1
  [VTQD_RDCActive_enum] -> VTQD_RDCActive_enum/1
  [VTQD_RegenMode_enum] -> VTQD_RegenMode_enum/1
  TorqueModule/66(VTQD_EEC2MSGCnt_raw) -> VTQD_EEC2MSGCnt_raw/1
  TorqueModule/67(VTQD_EEC2MSGCS_raw) -> VTQD_EEC2MSGCS_raw/1
  TorqueModule/68(VTQD_FDCCHAEBSRd4BRSta_enum) -> VTQD_FDCCHAEBSRd4BRSta_enum/1
  TorqueModule/69(VTQD_FDCCHAEBSHBSwSta_enum) -> VTQD_FDCCHAEBSHBSwSta_enum/1
  TorqueModule/70(VTQD_FDCCHAEBSHHSwSta_enum) -> VTQD_FDCCHAEBSHHSwSta_enum/1
  TorqueModule/71(VTQD_FDCVCUTUpAStaSta_enum) -> VTQD_FDCVCUTUpAStaSta_enum/1
  TorqueModule/72(VTQD_FDCVCUDACStatusSta_enum) -> VTQD_FDCVCUDACStatusSta_enum/1
  TorqueModule/73(VTQD_CoordTqDem_Nm) -> VTQD_CoordTqDem_Nm/1
  VTQR_RampREDUWhlTqReq_Nm/1 -> [VTQR_RampREDUWhlTqReq_Nm]
  [VTQR_RampREDUWhlTqReq_Nm] -> TorqueModule/57(VTQR_RampREDUWhlTqReq_Nm)
  TorqueModule/74(VTQD_FrEDUSpRat_rat) -> VTQD_FrEDUSpRat_rat/1
  TorqueModule/75(VTQD_RrEDUSpRat_rat) -> VTQD_RrEDUSpRat_rat/1
  VINP_EM1ReqTorqLimBrk_pct/1 -> [VINP_EM1ReqTorqLimBrk_pct]
  VINP_EM1ReqTorqLimDriv_pct/1 -> [VINP_EM1ReqTorqLimDriv_pct]
  VINP_EM1OvrCtrlMDriv_enum/1 -> [VINP_EM1OvrCtrlMDriv_enum]
  VINP_EM1OvrCtrlMBrk_enum/1 -> [VINP_EM1OvrCtrlMBrk_enum]
  [VINP_EM1ReqTorqLimBrk_pct] -> Signal_convert/25(VINP_EM1ReqTorqLimBrk_pct)
  [VINP_EM1ReqTorqLimDriv_pct] -> Signal_convert/26(VINP_EM1ReqTorqLimDriv_pct)
  [VINP_EM1OvrCtrlMBrk_enum] -> Signal_convert/27(VINP_EM1OvrCtrlMBrk_enum)
  [VINP_EM1OvrCtrlMDriv_enum] -> Signal_convert/28(VINP_EM1OvrCtrlMDriv_enum)
  Signal_convert/20(VTQD_EM1ReqTorqLimBrk_Nm) -> [VTQD_EM1ReqTorqLimBrk_Nm]
  Signal_convert/25(VTQD_EM1LimitCtrlDriv_flg) -> [VTQD_EM1LimitCtrlDriv_flg]
  Signal_convert/24(VTQD_EM1TorqueCtrlDriv_flg) -> [VTQD_EM1TorqueCtrlDriv_flg]
  Signal_convert/23(VTQD_EM1LimitCtrlBrk_flg) -> [VTQD_EM1LimitCtrlBrk_flg]
  Signal_convert/22(VTQD_EM1TorqueCtrlBrk_flg) -> [VTQD_EM1TorqueCtrlBrk_flg]
  Signal_convert/21(VTQD_EM1ReqTorqLimDriv_Nm) -> [VTQD_EM1ReqTorqLimDriv_Nm]
  [VTQD_EM1ReqTorqLimBrk_Nm] -> TorqueModule/58(VTQD_EM1ReqTorqLimBrk_Nm)
  [VTQD_EM1ReqTorqLimDriv_Nm] -> TorqueModule/59(VTQD_EM1ReqTorqLimDriv_Nm)
  [VTQD_EM1TorqueCtrlBrk_flg] -> TorqueModule/60(VTQD_EM1TorqueCtrlBrk_flg)
  [VTQD_EM1LimitCtrlBrk_flg] -> TorqueModule/61(VTQD_EM1LimitCtrlBrk_flg)
  [VTQD_EM1TorqueCtrlDriv_flg] -> TorqueModule/62(VTQD_EM1TorqueCtrlDriv_flg)
  [VTQD_EM1LimitCtrlDriv_flg] -> TorqueModule/63(VTQD_EM1LimitCtrlDriv_flg)
